simulink model "Propagator"  (R2020b)
settings: Solver=FixedStepAuto  StartTime=0.0  StopTime=sim_constants.simulation_time  FixedStep=sim_constants.time_step  RelTol=1e-3
undefined symbols (not defined in the file or in its folder): sim_constants
libraries: vrlib x2
settings Model: Creator=valerie  LastModifiedBy=newpo
settings DataIOCC: ReturnWorkspaceOutputs=off
settings DebuggingCC: ArithmeticOperatorsInVariantConditions=warning
settings SFSimCC: SimUseLocalCustomCode=off  CustomCodeUndefinedFunction=UseInterfaceOnly
settings RTWCC: RTWUseLocalCustomCode=off

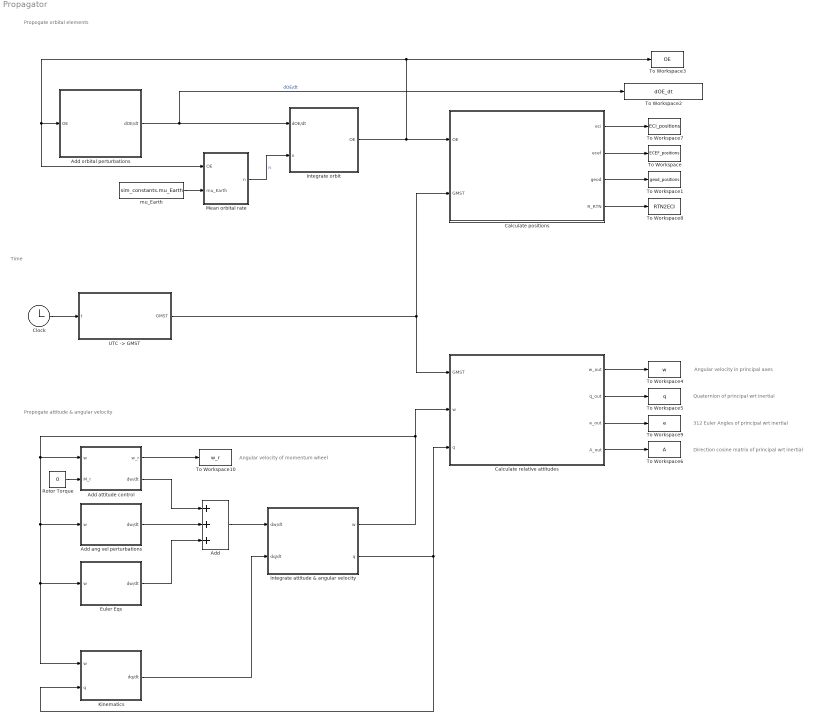
== system Propagator ==
  note: Angular velocity in principal axes
  note: Time
  note: Propogate orbital elements
  note: Propogate attitude & angular velocity
  note: Quaternion of principal wrt inertial
  note: Direction cosine matrix of principal wrt inertial
  note: 312 Euler Angles of principal wrt inertial
  note: Angular velocity of momentum wheel
  Add : Sum  Inputs=+++
  Add ang vel perturbations : Subsystem
  Add attitude control : Subsystem
  Add orbital perturbations : Subsystem
  Calculate positions : Subsystem
  Calculate relative attitudes : Subsystem
  Clock : Clock
  Euler Eqs : Subsystem
  Integrate attitude & angular velocity : Subsystem
  Integrate orbit : Subsystem
  Kinematics : Subsystem
  "Mean orbital rate " : MATLAB Function  TreatAsAtomicUnit=on
  Rotor Torque : Constant  Value=0
  To Workspace : ToWorkspace  VariableName=ECEF_positions  SaveFormat=Timeseries  SampleTime=-1
  To Workspace1 : ToWorkspace  VariableName=geod_positions  SaveFormat=Timeseries  SampleTime=-1
  To Workspace10 : ToWorkspace  VariableName=w_r  SaveFormat=Timeseries  SampleTime=-1
  To Workspace2 : ToWorkspace  VariableName=dOE_dt  SaveFormat=Timeseries  SampleTime=-1
  To Workspace3 : ToWorkspace  VariableName=OE  SaveFormat=Timeseries  SampleTime=-1
  To Workspace4 : ToWorkspace  VariableName=w  SaveFormat=Timeseries  SampleTime=-1
  To Workspace5 : ToWorkspace  VariableName=q  SaveFormat=Timeseries  SampleTime=-1
  To Workspace6 : ToWorkspace  VariableName=A  SaveFormat=Timeseries  SampleTime=-1
  To Workspace7 : ToWorkspace  VariableName=ECI_positions  SaveFormat=Timeseries  SampleTime=-1
  To Workspace8 : ToWorkspace  VariableName=RTN2ECI  SaveFormat=Timeseries  SampleTime=-1
  To Workspace9 : ToWorkspace  VariableName=e  SaveFormat=Timeseries  SampleTime=-1
  "UTC -> GMST" : MATLAB Function  TreatAsAtomicUnit=on
  mu_Earth : Constant  Value=sim_constants.mu_Earth
  wires:
  "UTC -> GMST"/1(GMST) -> Calculate relative attitudes/1(GMST), Calculate positions/2(GMST)
  Calculate positions/2(ecef) -> To Workspace/1
  Calculate positions/3(geod) -> To Workspace1/1
  mu_Earth/1 -> "Mean orbital rate "/2(mu_Earth)
  Add orbital perturbations/1(dOE/dt) -> To Workspace2/1, Integrate orbit/1(dOE/dt)  "dOE/dt"
  "Mean orbital rate "/1(n) -> Integrate orbit/2(n)  "n"
  Clock/1 -> "UTC -> GMST"/1(t)
  Integrate orbit/1(OE) -> "Mean orbital rate "/1(OE), Add orbital perturbations/1(OE), To Workspace3/1, Calculate positions/1(OE)
  Integrate attitude & angular velocity/1(w) -> Add attitude control/1(w), Add ang vel perturbations/1(w), Kinematics/1(w), Euler Eqs/1(w), Calculate relative attitudes/2(w)
  Add attitude control/2(dw/dt) -> Add/1
  Add ang vel perturbations/1(dw/dt) -> Add/2
  Add/1 -> Integrate attitude & angular velocity/1(dw/dt)
  Calculate relative attitudes/1(w_out) -> To Workspace4/1
  Integrate attitude & angular velocity/2(q) -> Kinematics/2(q), Calculate relative attitudes/3(q)
  Kinematics/1(dq/dt) -> Integrate attitude & angular velocity/2(dq/dt)
  Calculate relative attitudes/2(q_out) -> To Workspace5/1
  Calculate relative attitudes/4(A_out) -> To Workspace6/1
  Calculate positions/1(eci) -> To Workspace7/1
  Calculate positions/4(R_RTN) -> To Workspace8/1
  Calculate relative attitudes/3(e_out) -> To Workspace9/1
  Euler Eqs/1(dw/dt) -> Add/3
  Rotor Torque/1 -> Add attitude control/2(M_r)
  Add attitude control/1(w_r) -> To Workspace10/1

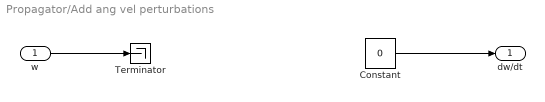
== system Propagator/Add ang vel perturbations ==
  w : Inport
  Constant : Constant  Value=0
  Terminator : Terminator
  dw/dt : Outport  VectorParamsAs1DForOutWhenUnconnected=off
  wires:
  w/1 -> Terminator/1
  Constant/1 -> dw/dt/1

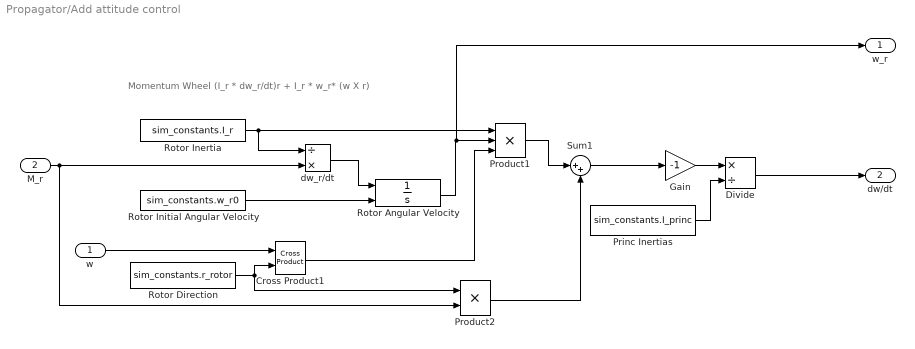
== system Propagator/Add attitude control ==
  note: Momentum Wheel (I_r * dw_r/dt)r + I_r * w_r* (w X r)
  w : Inport
  M_r : Inport  Port=2
  Cross Product1 : vrlib/Utilities/Cross Product
  Divide : Product  Inputs=*/
  Gain : Gain  Gain=-1
  Princ Inertias : Constant  Value=sim_constants.I_princ
  Product1 : Product  Inputs=3
  Product2 : Product
  Rotor Angular Velocity : Integrator  InitialConditionSource=external  LimitOutput=on  UpperSaturationLimit=sim_constants.w_rmax  LowerSaturationLimit=-sim_constants.w_rmax
  Rotor Direction : Constant  Value=sim_constants.r_rotor
  Rotor Inertia : Constant  Value=sim_constants.I_r
  Rotor Initial Angular Velocity : Constant  Value=sim_constants.w_r0
  Sum1 : Sum  Inputs=|++
  dw_r/dt : Product  Inputs=/*
  w_r : Outport  VectorParamsAs1DForOutWhenUnconnected=off
  dw/dt : Outport  Port=2  VectorParamsAs1DForOutWhenUnconnected=off
  wires:
  w/1 -> Cross Product1/1
  Gain/1 -> Divide/1
  Rotor Inertia/1 -> dw_r/dt/1, Product1/1
  Rotor Angular Velocity/1 -> w_r/1, Product1/2
  M_r/1 -> Product2/2, dw_r/dt/2
  Product1/1 -> Sum1/1
  dw_r/dt/1 -> Rotor Angular Velocity/1
  Rotor Initial Angular Velocity/1 -> Rotor Angular Velocity/2
  Rotor Direction/1 -> Product2/1, Cross Product1/2
  Sum1/1 -> Gain/1
  Divide/1 -> dw/dt/1
  Princ Inertias/1 -> Divide/2
  Product2/1 -> Sum1/2
  Cross Product1/1 -> Product1/3

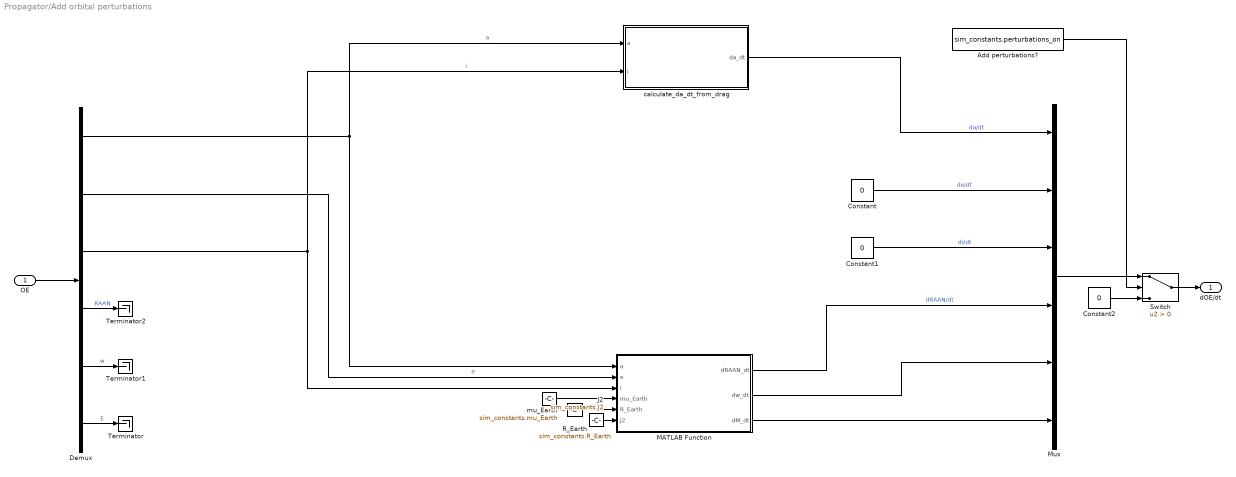
== system Propagator/Add orbital perturbations ==
  OE : Inport
  Add perturbations? : Constant  Value=sim_constants.perturbations_on
  Constant : Constant  Value=0
  Constant1 : Constant  Value=0
  Constant2 : Constant  Value=0
  Demux : Demux  Outputs=6
  J2 : Constant  Value=sim_constants.J2
  MATLAB Function : MATLAB Function  TreatAsAtomicUnit=on
  Mux : Mux  Inputs=6
  R_Earth : Constant  Value=sim_constants.R_Earth
  Switch : Switch  Criteria=u2 > Threshold
  Terminator : Terminator
  Terminator1 : Terminator
  Terminator2 : Terminator
  calculate_da_dt_from_drag : Subsystem
  mu_Earth : Constant  Value=sim_constants.mu_Earth
  dOE/dt : Outport  VectorParamsAs1DForOutWhenUnconnected=off
  wires:
  OE/1 -> Demux/1
  MATLAB Function/1(dRAAN_dt) -> Mux/4  "dRAAN/dt"
  Constant1/1 -> Mux/3  "di/dt"
  Constant/1 -> Mux/2  "de/dt"
  Mux/1 -> Switch/1
  Demux/6 -> Terminator/1  "E"
  Demux/5 -> Terminator1/1  "w"
  Demux/4 -> Terminator2/1  "RAAN"
  Demux/2 -> MATLAB Function/2(e)  "e"
  Demux/3 -> calculate_da_dt_from_drag/2(i), MATLAB Function/3(i)  "i"
  Demux/1 -> calculate_da_dt_from_drag/1(a), MATLAB Function/1(a)  "a"
  mu_Earth/1 -> MATLAB Function/4(mu_Earth)
  R_Earth/1 -> MATLAB Function/5(R_Earth)
  J2/1 -> MATLAB Function/6(J2)
  MATLAB Function/2(dw_dt) -> Mux/5
  MATLAB Function/3(dM_dt) -> Mux/6
  calculate_da_dt_from_drag/1(da_dt) -> Mux/1  "da/dt"
  Switch/1 -> dOE/dt/1
  Constant2/1 -> Switch/3
  Add perturbations?/1 -> Switch/2

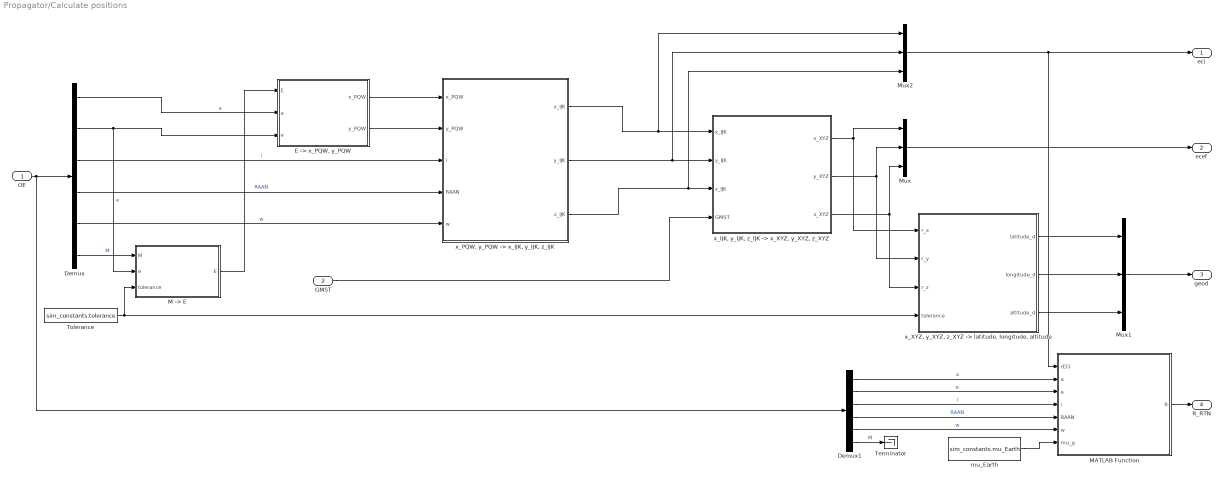
== system Propagator/Calculate positions ==
  OE : Inport
  GMST : Inport  Port=2
  " x_IJK, y_IJK, z_IJK -> x_XYZ, y_XYZ, z_XYZ" : MATLAB Function  TreatAsAtomicUnit=on
  " x_PQW, y_PQW -> x_IJK, y_IJK, z_IJK" : MATLAB Function  TreatAsAtomicUnit=on
  Demux : Demux  Outputs=6
  Demux1 : Demux  Outputs=6
  "E -> x_PQW, y_PQW" : MATLAB Function  TreatAsAtomicUnit=on
  "M -> E" : MATLAB Function  TreatAsAtomicUnit=on
  MATLAB Function : MATLAB Function  TreatAsAtomicUnit=on
  Mux : Mux  Inputs=3
  Mux1 : Mux  Inputs=3
  Mux2 : Mux  Inputs=3
  Terminator : Terminator
  Tolerance : Constant  Value=sim_constants.tolerance
  mu_Earth : Constant  Value=sim_constants.mu_Earth
  "x_XYZ, y_XYZ, z_XYZ -> latitude, longitude, altitude" : MATLAB Function  TreatAsAtomicUnit=on
  eci : Outport  VectorParamsAs1DForOutWhenUnconnected=off
  ecef : Outport  Port=2  VectorParamsAs1DForOutWhenUnconnected=off
  geod : Outport  Port=3  VectorParamsAs1DForOutWhenUnconnected=off
  R_RTN : Outport  Port=4  VectorParamsAs1DForOutWhenUnconnected=off
  wires:
  "E -> x_PQW, y_PQW"/2(y_PQW) -> " x_PQW, y_PQW -> x_IJK, y_IJK, z_IJK"/2(y_PQW)
  " x_PQW, y_PQW -> x_IJK, y_IJK, z_IJK"/1(x_IJK) -> Mux2/1, " x_IJK, y_IJK, z_IJK -> x_XYZ, y_XYZ, z_XYZ"/1(x_IJK)
  GMST/1 -> " x_IJK, y_IJK, z_IJK -> x_XYZ, y_XYZ, z_XYZ"/4(GMST)
  " x_PQW, y_PQW -> x_IJK, y_IJK, z_IJK"/3(z_IJK) -> Mux2/3, " x_IJK, y_IJK, z_IJK -> x_XYZ, y_XYZ, z_XYZ"/3(z_IJK)
  "E -> x_PQW, y_PQW"/1(x_PQW) -> " x_PQW, y_PQW -> x_IJK, y_IJK, z_IJK"/1(x_PQW)
  " x_IJK, y_IJK, z_IJK -> x_XYZ, y_XYZ, z_XYZ"/3(z_XYZ) -> Mux/3, "x_XYZ, y_XYZ, z_XYZ -> latitude, longitude, altitude"/3(r_z)
  " x_IJK, y_IJK, z_IJK -> x_XYZ, y_XYZ, z_XYZ"/2(y_XYZ) -> Mux/2, "x_XYZ, y_XYZ, z_XYZ -> latitude, longitude, altitude"/2(r_y)
  Mux1/1 -> geod/1
  Mux/1 -> ecef/1
  " x_IJK, y_IJK, z_IJK -> x_XYZ, y_XYZ, z_XYZ"/1(x_XYZ) -> Mux/1, "x_XYZ, y_XYZ, z_XYZ -> latitude, longitude, altitude"/1(r_x)
  Demux/5 -> " x_PQW, y_PQW -> x_IJK, y_IJK, z_IJK"/5(w)  "w"
  OE/1 -> Demux/1, Demux1/1
  Demux/2 -> "M -> E"/2(e), "E -> x_PQW, y_PQW"/3(e)  "e"
  Demux/4 -> " x_PQW, y_PQW -> x_IJK, y_IJK, z_IJK"/4(RAAN)  "RAAN"
  Demux/3 -> " x_PQW, y_PQW -> x_IJK, y_IJK, z_IJK"/3(i)  "i"
  Demux/1 -> "E -> x_PQW, y_PQW"/2(a)  "a"
  Tolerance/1 -> "M -> E"/3(tolerance), "x_XYZ, y_XYZ, z_XYZ -> latitude, longitude, altitude"/4(tolerance)
  Demux/6 -> "M -> E"/1(M)  "M"
  "M -> E"/1(E) -> "E -> x_PQW, y_PQW"/1(E)
  "x_XYZ, y_XYZ, z_XYZ -> latitude, longitude, altitude"/1(latitude_d) -> Mux1/1
  "x_XYZ, y_XYZ, z_XYZ -> latitude, longitude, altitude"/2(longitude_d) -> Mux1/2
  "x_XYZ, y_XYZ, z_XYZ -> latitude, longitude, altitude"/3(altitude_d) -> Mux1/3
  " x_PQW, y_PQW -> x_IJK, y_IJK, z_IJK"/2(y_IJK) -> Mux2/2, " x_IJK, y_IJK, z_IJK -> x_XYZ, y_XYZ, z_XYZ"/2(y_IJK)
  Mux2/1 -> eci/1, MATLAB Function/1(rECI)
  MATLAB Function/1(R) -> R_RTN/1
  mu_Earth/1 -> MATLAB Function/7(mu_g)
  Demux1/6 -> Terminator/1  "M"
  Demux1/5 -> MATLAB Function/6(w)  "w"
  Demux1/1 -> MATLAB Function/2(a)  "a"
  Demux1/2 -> MATLAB Function/3(e)  "e"
  Demux1/3 -> MATLAB Function/4(i)  "i"
  Demux1/4 -> MATLAB Function/5(RAAN)  "RAAN"

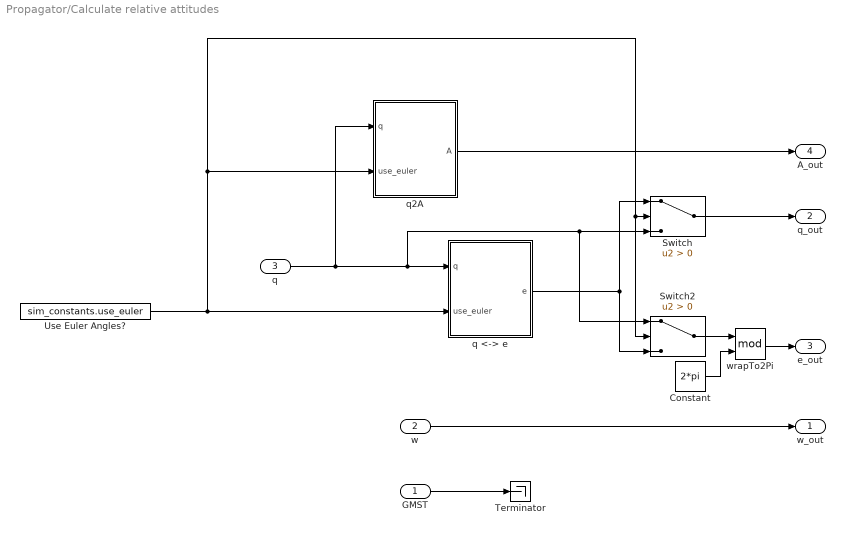
== system Propagator/Calculate relative attitudes ==
  GMST : Inport
  w : Inport  Port=2
  q : Inport  Port=3
  Constant : Constant  Value=2*pi
  Switch : Switch  Criteria=u2 > Threshold
  Switch2 : Switch  Criteria=u2 > Threshold
  Terminator : Terminator
  Use Euler Angles? : Constant  Value=sim_constants.use_euler
  q <-> e : MATLAB Function  TreatAsAtomicUnit=on
  q2A : MATLAB Function  TreatAsAtomicUnit=on
  wrapTo2Pi : Math  Operator=mod  SaturateOnIntegerOverflow=on
  w_out : Outport  VectorParamsAs1DForOutWhenUnconnected=off
  q_out : Outport  Port=2  VectorParamsAs1DForOutWhenUnconnected=off
  e_out : Outport  Port=3  VectorParamsAs1DForOutWhenUnconnected=off
  A_out : Outport  Port=4  VectorParamsAs1DForOutWhenUnconnected=off
  wires:
  w/1 -> w_out/1
  GMST/1 -> Terminator/1
  q/1 -> q2A/1(q), q <-> e/1(q), Switch2/1, Switch/3
  Switch/1 -> q_out/1
  q2A/1(A) -> A_out/1
  Switch2/1 -> wrapTo2Pi/1
  Use Euler Angles?/1 -> q2A/2(use_euler), Switch2/2, Switch/2, q <-> e/2(use_euler)
  q <-> e/1(e) -> Switch2/3, Switch/1
  wrapTo2Pi/1 -> e_out/1
  Constant/1 -> wrapTo2Pi/2

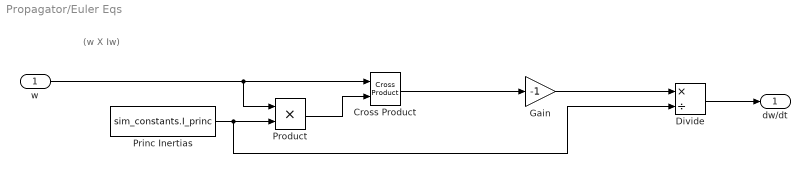
== system Propagator/Euler Eqs ==
  note: (w X Iw)
  w : Inport
  Cross Product : vrlib/Utilities/Cross Product
  Divide : Product  Inputs=*/
  Gain : Gain  Gain=-1
  Princ Inertias : Constant  Value=sim_constants.I_princ
  Product : Product
  dw/dt : Outport
  wires:
  Princ Inertias/1 -> Product/2, Divide/2
  w/1 -> Cross Product/1, Product/1
  Product/1 -> Cross Product/2
  Cross Product/1 -> Gain/1
  Gain/1 -> Divide/1
  Divide/1 -> dw/dt/1

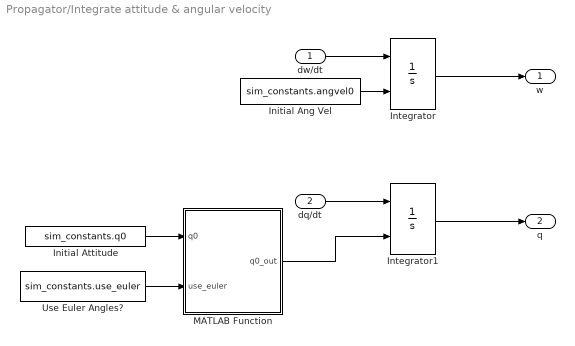
== system Propagator/Integrate attitude & angular velocity ==
  dw/dt : Inport
  dq/dt : Inport  Port=2
  Initial Ang Vel : Constant  Value=sim_constants.angvel0
  Initial Attitude : Constant  Value=sim_constants.q0
  Integrator : Integrator  InitialConditionSource=external
  Integrator1 : Integrator  InitialConditionSource=external
  MATLAB Function : MATLAB Function  TreatAsAtomicUnit=on
  Use Euler Angles? : Constant  Value=sim_constants.use_euler
  w : Outport
  q : Outport  Port=2
  wires:
  Integrator/1 -> w/1
  dw/dt/1 -> Integrator/1
  Initial Ang Vel/1 -> Integrator/2
  dq/dt/1 -> Integrator1/1
  Initial Attitude/1 -> MATLAB Function/1(q0)
  Integrator1/1 -> q/1
  Use Euler Angles?/1 -> MATLAB Function/2(use_euler)
  MATLAB Function/1(q0_out) -> Integrator1/2

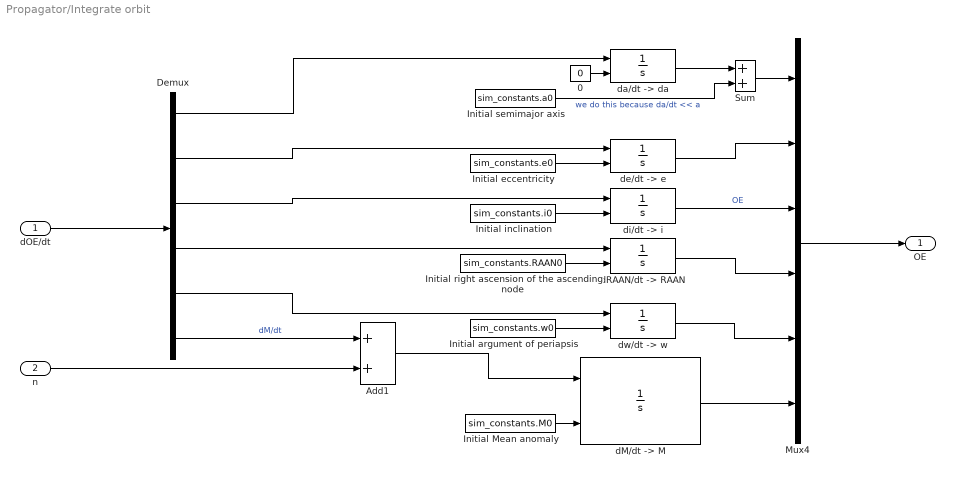
== system Propagator/Integrate orbit ==
  dOE/dt : Inport
  n : Inport  Port=2
  0 : Constant  Value=0
  Add1 : Sum
  Demux : Demux  Outputs=6
  Initial Mean anomaly : Constant  Value=sim_constants.M0
  Initial argument of periapsis : Constant  Value=sim_constants.w0
  Initial eccentricity : Constant  Value=sim_constants.e0
  Initial inclination : Constant  Value=sim_constants.i0
  Initial right ascension of the ascending node : Constant  Value=sim_constants.RAAN0
  Initial semimajor axis : Constant  Value=sim_constants.a0
  Mux4 : Mux  Inputs=6
  Sum : Sum
  "dM/dt -> M" : Integrator  InitialConditionSource=external  WrapState=on  WrappedStateUpperValue=2*pi  WrappedStateLowerValue=0
  "dRAAN/dt -> RAAN" : Integrator  InitialConditionSource=external  WrappedStateUpperValue=180  WrappedStateLowerValue=0
  "da/dt -> da" : Integrator  InitialConditionSource=external
  "de/dt -> e" : Integrator  InitialConditionSource=external
  "di/dt -> i" : Integrator  InitialConditionSource=external  WrapState=on  WrappedStateUpperValue=180  WrappedStateLowerValue=0
  "dw/dt -> w" : Integrator  InitialConditionSource=external  WrapState=on  WrappedStateUpperValue=360  WrappedStateLowerValue=0
  OE : Outport  VectorParamsAs1DForOutWhenUnconnected=off
  wires:
  Mux4/1 -> OE/1
  dOE/dt/1 -> Demux/1
  Demux/6 -> Add1/1  "dM/dt"
  Demux/5 -> "dw/dt -> w"/1
  Initial inclination/1 -> "di/dt -> i"/2
  n/1 -> Add1/2
  Add1/1 -> "dM/dt -> M"/1
  "dM/dt -> M"/1 -> Mux4/6
  "di/dt -> i"/1 -> Mux4/3  "OE"
  Demux/3 -> "di/dt -> i"/1
  Demux/1 -> "da/dt -> da"/1
  Demux/2 -> "de/dt -> e"/1
  Initial eccentricity/1 -> "de/dt -> e"/2
  Initial argument of periapsis/1 -> "dw/dt -> w"/2
  Initial right ascension of the ascending node/1 -> "dRAAN/dt -> RAAN"/2
  "dRAAN/dt -> RAAN"/1 -> Mux4/4
  Demux/4 -> "dRAAN/dt -> RAAN"/1
  "dw/dt -> w"/1 -> Mux4/5
  Initial Mean anomaly/1 -> "dM/dt -> M"/2
  "de/dt -> e"/1 -> Mux4/2
  Initial semimajor axis/1 -> Sum/2  "we do this because da/dt << a"
  0/1 -> "da/dt -> da"/2
  Sum/1 -> Mux4/1
  "da/dt -> da"/1 -> Sum/1

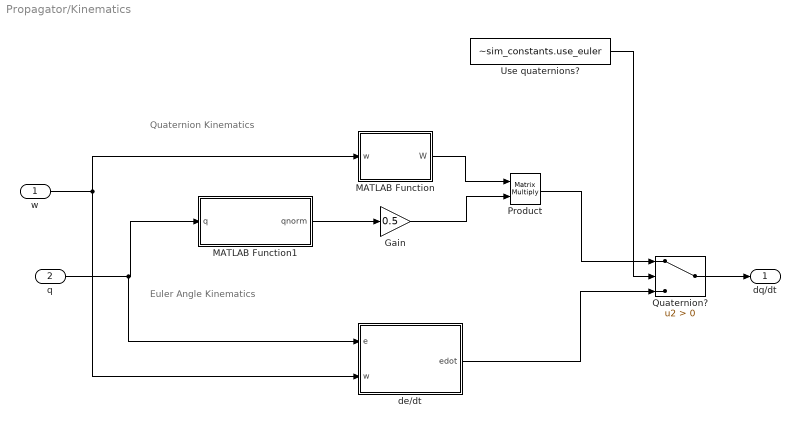
== system Propagator/Kinematics ==
  note: Euler Angle Kinematics
  note: Quaternion Kinematics
  w : Inport
  q : Inport  Port=2
  Gain : Gain  Gain=0.5
  MATLAB Function : MATLAB Function  TreatAsAtomicUnit=on
  MATLAB Function1 : MATLAB Function  TreatAsAtomicUnit=on
  Product : Product  Multiplication=Matrix(*)
  Quaternion? : Switch  Criteria=u2 > Threshold
  Use quaternions? : Constant  Value=~sim_constants.use_euler
  de/dt : MATLAB Function  TreatAsAtomicUnit=on
  dq/dt : Outport
  wires:
  Gain/1 -> Product/2
  w/1 -> MATLAB Function/1(w), de/dt/2(w)
  MATLAB Function/1(W) -> Product/1
  MATLAB Function1/1(qnorm) -> Gain/1
  Quaternion?/1 -> dq/dt/1
  Product/1 -> Quaternion?/1
  Use quaternions?/1 -> Quaternion?/2
  de/dt/1(edot) -> Quaternion?/3
  q/1 -> de/dt/1(e), MATLAB Function1/1(q)

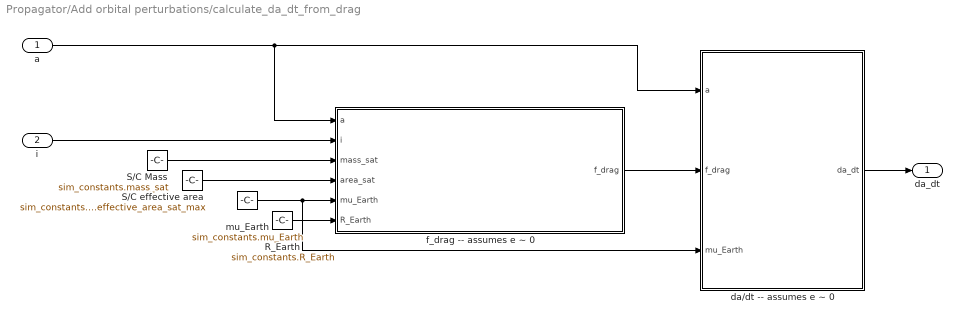
== system Propagator/Add orbital perturbations/calculate_da_dt_from_drag ==
  a : Inport
  i : Inport  Port=2
  R_Earth : Constant  Value=sim_constants.R_Earth
  S/C Mass : Constant  Value=sim_constants.mass_sat
  S/C effective area : Constant  Value=sim_constants.effective_area_sat_max
  "da/dt -- assumes e ~ 0" : MATLAB Function  TreatAsAtomicUnit=on
  "f_drag -- assumes e ~ 0" : MATLAB Function  TreatAsAtomicUnit=on
  mu_Earth : Constant  Value=sim_constants.mu_Earth
  da_dt : Outport  VectorParamsAs1DForOutWhenUnconnected=off
  wires:
  mu_Earth/1 -> "f_drag -- assumes e ~ 0"/5(mu_Earth), "da/dt -- assumes e ~ 0"/3(mu_Earth)
  "f_drag -- assumes e ~ 0"/1(f_drag) -> "da/dt -- assumes e ~ 0"/2(f_drag)
  "da/dt -- assumes e ~ 0"/1(da_dt) -> da_dt/1
  S/C Mass/1 -> "f_drag -- assumes e ~ 0"/3(mass_sat)
  S/C effective area/1 -> "f_drag -- assumes e ~ 0"/4(area_sat)
  a/1 -> "f_drag -- assumes e ~ 0"/1(a), "da/dt -- assumes e ~ 0"/1(a)
  R_Earth/1 -> "f_drag -- assumes e ~ 0"/6(R_Earth)
  i/1 -> "f_drag -- assumes e ~ 0"/2(i)

== matlab function Propagator/Add orbital perturbations/calculate_da_dt_from_drag/da//dt -- assumes e ~ 0 ==
  data: a input; f_drag input; da_dt output; mu_Earth input
function da_dt = calculate_da_dt_from_drag(a, f_drag, mu_Earth)
    % Calculates the effect of drag on the orbit's a in km/sec given
    % a (in km) and f_drag (in km/s). Assumes e ~ 0.
    
    n = (mu_Earth/(a^3))^(1/2); % s-1
    
    % e ~ 0 -> drag force is entirely in T
    da_dt = (2/n)*f_drag; % km s-1
    
end

== matlab function Propagator/Add orbital perturbations/calculate_da_dt_from_drag/f_drag -- assumes e ~ 0 ==
  data: a input; i input; mass_sat input; area_sat input; mu_Earth input; R_Earth input; f_drag output
function f_drag = calculate_atmospheric_drag_acceleration(a, i, ...
    mass_sat, area_sat, mu_Earth, R_Earth)
    % Calculate the acceleration (in km/sec^2) on a satellite due to 
    % atmospheric drag, given the satellite's mass, area, semimajor axis, 
    % and inclination.

    % Constants
    w_Earth = 7.29*10^-5; % rad s-1
    C_D = 2.3;  % empirical, unitless
    
    % Drag (ballistic) coefficient
    B = (C_D*area_sat/mass_sat)/(1000^2); % m2 kg-1 -> km2 kg-1 
    
    % Atmospheric density
    % From http://www.braeunig.us/space/atmos.htm
    % Density @ reference altitude h0 = 550km
    rho_0 = (2.14*10^-13)*(1000^3); % kg m-3 -> kg km-3, 
    h0 = 550 + R_Earth; % km, reference altitude -> radius
    H = 68.7; % km, atmospheric scale height
    
    rho = rho_0*exp(-(a-h0)/H); % kg km-3
    
    % Velocities. Because e~0, velocities are entirely in T
    v_air = w_Earth*a*cosd(i); % km s-1 
    v_orbital = sqrt(mu_Earth/a); % km s-1 
    
    v_rel = v_orbital - v_air;    % km s-1
    
    % The actual drag
    f_drag = - (B*rho*v_rel^2)/2; % km s-2

end

== matlab function Propagator/Kinematics/MATLAB Function ==
  data: w input; W output
function W = make_Omega(w)
    W = [   0     w(3)  -w(2)  w(1); 
           -w(3)  0     w(1)   w(2);
            w(2) -w(1)   0     w(3);
           -w(1) -w(2)  -w(3)  0    ] ; 
end

== matlab function Propagator/Calculate positions/MATLAB Function ==
  data: rECI input; a input; e input; i input; RAAN input; w input; R output; mu_g input
%% OE2RTN -
% Takes in orbital elements and spits out the rotation matrix from RTN frame
% to ECI. 
function R = OE2RTN(rECI,a,e,i,RAAN, w,mu_g)
    R = zeros(3,3);
    if e == 0 % protect against circular orbit (undefined w)
       w = 0; 
    end
    if i == 0 % protect against equatorial orbit (undefined i)
       RAAN = 0; 
    end
    %Calculate additional useful orbit parameters
    p = a*(1-e^2);
    h = sqrt(mu_g * p);
    
    %Calculate position and velocity vectors
    rotm = rotz(-RAAN)*rotx(-i)*rotx(-w);
        % ... Rotation matrix from PQW to IJK 
    hECI = (rotm*([0;0;h])); % rotate ang momentum from PQW to IJK
    R(:,1) = rECI/norm(rECI); % normalize radial vector
    R(:,3) = hECI/norm(hECI); % parallel to angular momentum
    R(:,2) = cross(R(:,3),R(:,1)); % T completes the right-handed triad
end

== matlab function Propagator/Kinematics/MATLAB Function1 ==
  data: q input; qnorm output
function qnorm = normalize_quaternion(q)
    qnorm = q./norm(q);
end

== matlab function Propagator/Calculate relative attitudes/q2A ==
  data: q input; A output; use_euler input
%% q2A - Calculate cosine matrix from q (or euler angles)
function A = toCosineMatrix(q, use_euler)
    if ~use_euler
        qvec = reshape(q(1:3),3,1);
        skewq = [0 -qvec(3) qvec(2); qvec(3) 0 -qvec(1) ; -qvec(2) qvec(1) 0];
        A = (q(4)^2 - sum(qvec.^2))*eye(3) + 2*qvec*(qvec') - 2*q(4)*skewq ;
    else
        A = [cos(q(1))*cos(q(3))+prod(sin(q(1:3))) sin(q(1))*cos(q(2)) -cos(q(1))*sin(q(3))+sin(q(1))*sin(q(2))*cos(q(3)); 
             (-sin(q(1))*cos(q(3))+cos(q(1))*sin(q(2))*sin(q(3))) (cos(q(1))*cos(q(2))) sin(q(1))*sin(q(3))+cos(q(1))*sin(q(2))*cos(q(3));
             cos(q(2))*sin(q(3)) -sin(q(2)) cos(q(2))*cos(q(3)) ];
        A = A';
    end
end

== matlab function Propagator/Integrate attitude & angular velocity/MATLAB Function ==
  data: q0 input; q0_out output; use_euler input
%% q2e - Calculate 312 euler angles from quaternion
function q0_out = q2e(q0, use_euler)
    if ~use_euler
        % If quaternions, q0 is already in appropriate format
        q0_out = q0;
    else
        % If using euler angles, transform quaternion to 312 Euler
        % euler = [phi, theta, psi]
        q0_out = zeros(4,1); q0 = q0/norm(q0);
        q0_out(1) = atan2(2*q0(1)*q0(2)+ 2*q0(4)*q0(3),q0(2)^2-q0(3)^2+q0(4)^2-q0(1)^2);
        q0_out(2) = -asin(2*q0(2)*q0(3)-2*q0(4)*q0(1));
        q0_out(3) = atan2(2*q0(1)*q0(3)+ 2*q0(4)*q0(2),-q0(2)^2+q0(3)^2+q0(4)^2-q0(1)^2);
        q0_out(4) = 0; % just a place holder for constant size
    end
end

== matlab function Propagator/Kinematics/de//dt ==
  data: e input; edot output; w input
function edot = euler312_rate(e,w)
    edot = zeros(size(e));
    edot(1) = (w(1)*sin(e(3))+w(3)*cos(e(3)))/cos(e(2));
    edot(2) = w(1)*cos(e(3)) - w(3)*sin(e(3));
    edot(3) = w(2) - tan(e(2))*(w(1)*sin(e(3)) + w(3)*cos(e(3)));
end

== matlab function Propagator/Calculate relative attitudes/q <-> e ==
  data: q input; e output; use_euler input
%% q_backforth_e - Calculate 312 euler angles from quaternion (or vice versa)
function e = q_backforth_e(q, use_euler)
    if ~use_euler
        % If quaternions, calculate 312 angles from q
        e = zeros(4,1); q = q/norm(q); 
        e(1) = atan2(2*q(1)*q(2)+ 2*q(4)*q(3),q(2)^2-q(3)^2+q(4)^2-q(1)^2);
        e(2) = -asin(2*q(2)*q(3)-2*q(4)*q(1));
        e(3) = atan2(2*q(1)*q(3)+ 2*q(4)*q(2),q(3)^2-q(2)^2-q(1)^2+q(4)^2);
        e(4) = 0;
    else
        % If euler angles, calculate quaternion
        % euler = [phi, theta, psi]
        q = q/2;
        e = zeros(4,1);
        e(1) = prod(cos(q(1:3))) + prod(sin(q(1:3)));
        e(2) = cos(q(1))*sin(q(2))*cos(q(3)) + sin(q(1))*cos(q(2))*sin(q(3));
        e(3) = cos(q(1))*cos(q(2))*sin(q(3)) + sin(q(1))*sin(q(3))*cos(q(2));
        e(4) = -cos(q(1))*sin(q(2))*sin(q(3)) + sin(q(1))*cos(q(2))*cos(q(3));
    end
end

== matlab function Propagator/Calculate positions/E -> x_PQW, y_PQW ==
  data: E input; a input; x_PQW output; e input; y_PQW output
function [x_PQW, y_PQW] = E2perifocal(E,a,e)
    % Given an eccentric anomaly E and orbital eccentricity e, calculates 
    % the perifocal coordinates (x_PQW, y_PQW)
    
    x_PQW = a*(cos(E) - e);
    y_PQW = a*sqrt(1-e^2)*sin(E);

== matlab function Propagator/Calculate positions/M -> E ==
  data: M input; E output; e input; tolerance input
function E = mean2eccentric(M, e, tolerance)
    % Given the mean anomaly M (in rad), eccentricity e, and tolerance, 
    % calculates the eccentric anomaly E (in rad) using the Newton-Raphson
    % method.
    
    % Initialize N-R
    E = M;
    d = calculate_new_delta(E, M, e);
    
    while abs(d) >= tolerance
        E = E + d;
        d = calculate_new_delta(E, M, e);
    end
end

function d = calculate_new_delta(E, M, e)
    % Calculates a new delta d to be used for calculating the eccentric 
    % anomaly E (in rad) using the Newton-Raphson method.
    
    d = -(E - e*sin(E) - M)/(1 - e*cos(E));
end

function M = eccentric2mean(E, e)
    % Given an eccentric anomaly E and orbital eccentricity e, calculates 
    % the mean anomaly M (in rad).

    M = E - e*sin(E);
end

== matlab function Propagator/Calculate positions/ x_PQW, y_PQW -> x_IJK, y_IJK, z_IJK ==
  data: x_PQW input; y_PQW input; x_IJK output; y_IJK output; z_IJK output; i input; RAAN input; w input
function [x_IJK, y_IJK, z_IJK] = perifocal2ECI(x_PQW, y_PQW, i, RAAN, w)
    % Given perifocal coordinates (x_PQW, y_PQW) and a subset of the 
    % Keplerian orbit elements (i, RAAN, w [in deg]), calculates ECI
    % coordinates (x_IJK, y_IJK, z_IJK).
    
    % By definition
    z_PQW = 0;
    
    r_IJK = calculate_pqw_R_ijk(i, RAAN, w)*[x_PQW, y_PQW, z_PQW]';
    
    x_IJK = r_IJK(1);
    y_IJK = r_IJK(2);
    z_IJK = r_IJK(3);

end 

function pqw_R_ijk = calculate_pqw_R_ijk(i, RAAN, w)
    % Calculates rotation matrix that tranforms position and velocity in 
    % PQW coordinates (r_PQW) to ECI coordinates (r_ECI) given a
    % subset of the Keplerian orbit elements (i, RAAN, w) [in rad] 

        pqw_R_ijk = rotz(-RAAN)*rotx(-i)* ...
            rotx(-w);
end

== matlab function Propagator/Calculate positions/ x_IJK, y_IJK, z_IJK -> x_XYZ, y_XYZ, z_XYZ ==
  data: x_IJK input; y_IJK input; z_IJK input; x_XYZ output; y_XYZ output; z_XYZ output; GMST input size=1
function [x_XYZ, y_XYZ, z_XYZ] = ECI2ECEF(x_IJK, y_IJK, z_IJK, GMST)
    % Given Earth-centered inertial coordinates (x_IJK, y_IJK, z_IJK),
    % and the Greenwich Meridian Standard Time, calculates Earth-centered,
    % Earth-fixed coordinates (x_XYZ, y_XYZ, z_XYZ).
    
    r_XYZ = crf2trf(GMST)* ...
        [x_IJK, y_IJK, z_IJK]';
    
    x_XYZ = r_XYZ(1);
    y_XYZ = r_XYZ(2);
    z_XYZ = r_XYZ(3);

end 

function rot = crf2trf(gmst)
    % I did not complete Homework 4, so this function is copied + pasted
    % from the solutions.
    % Creates a rotation matrix between CRF and TRF systems
    % Inputs:
    %   gmst - Greenwich Mean Sidereal Time [rad]
    % Outputs:
    %   rot - rotation matrix from celestial to terrestrial
    %   reference frames
    
    rot = rotz(rad2deg(-gmst));
end

== matlab function Propagator/UTC -> GMST ==
  data: GMST output size=1; t input
function GMST = convert_time(t)
    % Converts time to GMST for orbital propagation. 
    
    % Propagate time
    mj_day = t/(24*3600);
    
    GMST = mj_day2GMST(mj_day);   
    
end

function GMST = mj_day2GMST(modified_julian_day)
    % Converts UT1 time in MJD to GMST (in rad).
    
    % Normalize by epoch (Jan. 1, 2000 12:00 h)
    d = modified_julian_day - 51544.5;
    
    GMST_deg = 280.4606 + 360.9856473*d; 
    GMST = mod(deg2rad(GMST_deg), 2*pi);

end

== matlab function Propagator/Calculate positions/x_XYZ, y_XYZ, z_XYZ -> latitude, longitude, altitude ==
  data: latitude_d output; longitude_d output; r_x input; r_y input; altitude_d output; r_z input; tolerance input
function [latitude_d, longitude_d, altitude_d] = ... 
    ECEF2geod(r_x, r_y, r_z, tolerance)
% Calculates geodetic coordinates (altutude_d, latitude_d, longitude_d) 
% [deg] given ECEF coordinates (r_x, r_y, r_z) and some tolerance.
    
    % Constants
    R_E = 6378;     % km
    e_E = 0.0818;   % unitless
    
    r_xy = norm([r_x, r_y]);

    % Initialize N-R
    [latitude_d, longitude_d, altitude_d] = ECEF2geoc(r_x, r_y, r_z);
    error = tolerance + 0.01;
    N = R_E;
    
    while abs(error) > tolerance
        old_latitude_d = latitude_d;
        
        % Radius of curvature, km
        N = R_E/sqrt(1 - e_E^2*sind(latitude_d)^2);
        
        % Update geodetic latitude
        latitude_d = atan2d(r_z + N*e_E^2*sind(old_latitude_d), r_xy);
        error = latitude_d - old_latitude_d;
    end
    
    % Finally, height above ellipsoid
    altitude_d = r_xy/cosd(latitude_d) - N;

end

function [latitude_c, longitude_c, altitude_c] = ECEF2geoc(r_x, r_y, r_z)
% Calculates geocentric coordinates (altutude_c, latitude_c, _clongitude) 
% [deg] given ECEF coordinates (r_x, r_y, r_z).
    
    % Constants
    R_Earth = 6371; % km

    r = norm([r_x, r_y, r_z]); % km
    
    latitude_c = asind(r_z/r);        % deg
    longitude_c = atan2d(r_y, r_x);   % deg
    altitude_c = r - R_Earth;         % km

end

== matlab function Propagator/Mean orbital rate  ==
  data: OE input; n output; mu_Earth input
function n = calculate_n(OE, mu_Earth)
    % Given a semimajor axis a, calculates the mean orbital rate n 
    % (in rad/s).
    
    a = OE(1);
    
    n = sqrt(mu_Earth/a^3);
    
end

== matlab function Propagator/Add orbital perturbations/MATLAB Function ==
  data: a input; dRAAN_dt output; e input; i input; mu_Earth input; R_Earth input; J2 input; dw_dt output; dM_dt output
function [dRAAN_dt, dw_dt, dM_dt] = calculate_dOE_dt_from_J2(a, e, i, ...
    mu_Earth, R_Earth, J2)
    % Calculates the effect of J2 on the orbit's RAAN, w, and M in deg/sec. 
    % given a (in km), e, and i (in deg). 
    % If 0 < i < 90, then dRAAN/dt < 0; if 90 < i < 180, dRAAN/dt > 0.
    % If 0 < i < 63.43, then dw/dt > 0; if 63.43 < i < 116.6, dw/dt < 0.
    % If 0 < i < 63.43, then dw/dt > 0; if 63.43 < i < 116.6, dw/dt < 0.
    
    % Common coefficient for all three dOE/dt
    n = ((a^3)/mu_Earth)^-(1/2);
    coefficient = n * J2 * ( R_Earth / (a*(1-e^2)) )^2;
    
    dRAAN_dt = rad2deg( -(3/2) * coefficient * cosd(i) );
    
    dw_dt = rad2deg( (3/4) * coefficient * (5*(cosd(i)^2) - 1) );

    % Removed + n in equations from lecture notes as that is summed 
    % before the integrator elsewhere
    dM_dt = rad2deg( (3/4) * coefficient * sqrt(1-e^2) * ...
        (3*(cosd(i)^2) - 1) );;
    
end
